simulink model "Week3_Problem2"  (R2020b)
settings: Solver=VariableStepAuto  StartTime=0.0  StopTime=10.0  RelTol=1e-3
settings Model: Creator=ASUS  LastModifiedBy=ASUS

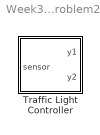
== system Week3_Problem2 ==
  "Traffic Light Controller " : Stateflow chart  TreatAsAtomicUnit=on

== stateflow chart Week3_Problem2/Traffic Light Controller  ==
  note: Traffic Light Controller by Moore Model
      |
      | Lets assume that the traffic in North-South is higher than that of at East-West. So the Green light for North-South path will be high
  note: Stop State
      | Output y1 is set to Red in the East-West side.
      | Output y2 is set to Green in the North-South side.
      | After 30 ticks the state will change to Stop_For_Traffic State
  state Stop
    y1=Red;
    y2=Green;
  state Stop_for_Traffic
    y1=Red;
    y2=Green;
  state Stop_to_Go
    y1=Red;
    y2=Yellow;
  note: Stop_for_Traffic State
      | Output y1 is set to Red in the East-West side.
      | Output y2 is set to Green in the North-South side.
      | Checks the signal sensor.
      | If the sensor signal is true then the cars are waiting East-West Side
      | then the state changed to Stop_to_Go
  state Go_to_Stop
    y1=Yellow;
    y2=Red;
  state Go
    y1=Green;
    y2=Red;
  note: Stop_to_Go
      | Output y1 is set to Red in the East-West side.
      | Output y2 is set to Yellow in the North-South side.
      | After 3 tick the state changes to Go.
  note: Go
      | Output y1 is set Green in the East-West side.
      | Output y2 is set to Red in the North-South side.
      | After 15 tick the state changes to Go_to_Stop
  note: Go_to_Stop
      | Output y1 is set Yellow in the East-West side.
      | Output y2 is set to Red in the North-South side.
      | After 3 tick the state changes to Stop
  (default) -> Stop
  Stop_for_Traffic -> Stop_to_Go : [sensor]
  Stop -> Stop_for_Traffic : after(30,tick)
  Go_to_Stop -> Stop : after(3,tick)
  Stop_to_Go -> Go : after(3,tick)
  Go -> Go_to_Stop : after(15,tick)
  data: y1 output; y2 output; Red constant double; Yellow constant double; Green constant double; sensor input
